simulink model "BiT_Template_pavlo"  (R2025b)
settings: Solver=ode3  StartTime=0.0  StopTime=30  FixedStep=0.005  RelTol=1e-3
StopFcn:
  | user_confirmed = true;
  | disp('Gestoppt?!')
  | 
  | % stop(t);
  | % delete(t);
  | 
  | %% Switch to Config Mode
  | %Tc3_AI.sysManager.ActivateConfiguration();
  | %
  | % Tc3_AI.SwitchToConfig('local')
  | %
  | % %save Solution
  | % Tc3_AI.SaveSolution();
  | %
  | % %% Close Aktive VS Instance
  | % Tc3_AI.closeVsInstance();
libraries: slpidlib x1
settings Model: Creator=clemensm  LastModifiedBy=Felix
settings OptimizationCC: LocalBlockOutputs=off
settings RTWCC: SystemTargetFile=TwinCatGrt.tlc  GenCodeOnly=on  GenerateMakefile=off  TemplateMakefile=tcgrt_msbuild.tmf  TargetLang=C++  Description=TwinCAT GRT Target
settings STFCustomTargetCC: SystemTargetFile=TwinCatGrt.tlc  TargetLangStandard=C++11 (ISO)  CombineOutputUpdateFcns=on  CodeInterfacePackaging=Reusable function  CPPClassGenCompliant=on  GRTInterface=off  GenerateAllocFcn=on  TcCom_DWorkReadOnly=on  TcProject_StaticStlStringCapacity=Auto  TcPlcFb_MonitorExecutionTime=off  TcCom_ContStateCreateSymbols=on  TcProject_IgnorePseudoArrayDimensions=off  TcProject_IncrementVersion=Revision  TcProject_DeployRestart=off  TcProject_UseCodeInfoExporter=on  TcProject_CLanguageStandard=Default  TcCom_VariableSymbolMapping=Identical  TcProject_DrvFileVersion=$<VersionFromFile>  TcProject_ProjectDir=C:\TwinCAT\3.1\CustomConfig\Modules\Ctrl_only  TcProject_DrvProductVersion=$<DrvFileVersion>  TcPlcFb_OemLicenses=$<Project:OemLicenses>  TcCom_OutputCreateSymbols=on  TcCom_TcComWrapperFbProperties=off  TcProject_UseStaticStlString=off  TcProject_PublishTcOSARMv7M=off  TcCom_OnlineChangeRestoreDataAreas=off  TcCom_AllowDataAreaForSharedData=off  TcProject_LibCatPath=$<Project:Dir>\$<Project:Name>.libcat.xml  TcCom_OemLicenses=$<Project:OemLicenses>  TcProject_UseIntrinsics=on  TcCom_ExtendSignalResolution=on  TcCom_ExtModeRtAllowForParameterChange=on  TcProject_UseCodeDescriptor=on  TcProject_SignWithTwinCatCertificate=inherit default  TcProject_GeneratePlcLibrary=off  TcProject_PublishTcOSARMv7A=off  TcProject_PreferIntOverLong=off  TcPlcFb_ExtModeRtAllowExecutionCommands=off  TcProject_Generate=on  TcProject_GenerateStructDutsWithDefaultValues=Auto  TcCom_ExecutionInfoParam=on  TcCom_TcComWrapperFb=off  TcCom_Generate=on  TcProject_PublishParallel=on  TcCom_OutputDataAccess=Output Source DataArea  TcProject_CppLanguageStandard=Default  TcCom_ParametersCreateSymbols=on  TcProject_PublishTcRTx86=on  TcCom_ExecuteModelCode=on  TcPlcFb_UpdateExceptionHandling=CallerExceptions  TcProject_PublishTcRTx64=on  TcCom_OriginalIoBlockNames=off  TcProject_SignTwinCatCertName=MCI_2024_OEM.tccert  TcCom_InputReadOnly=off  TcCom_GroupDisplayName=$<GroupName>  TcProject_PlcVarPrefixes=PVOID=p | BOOL=b | BOOL32=b | DATE=d | TIME_OF_DATE=td | TIME=t | LTIME=t | GUID=n  TcCom_GlobalParamDefaultSharing=Define  TcCom_MonitorExecutionTime=off  TcProject_VersionSrc=$<LatestTMFile>  TcCom_ExecutionSequence=UpdateBeforeOutputMapping  TcCom_InputCreateSymbols=on  TcProject_DataExchangeModulesVersion=$<ModuleGenerator:DataExchange:Version>  TcCom_BlockDiagramVariableAccess=AssignToParent  TcCom_GroupIcon=$<TE140x:Icon>  TcCom_ParametersDataAccess=Internal DataArea  TcProject_LibraryCategories=$<VendorName>  TcProject_CreateUniqueEnumItemNames=off  TcProject_PreferToolArchitectureX64=on  TcProject_PublishPlatformtoolset=Auto  TcCom_InputInitValues=off  TcProject_Description=TwinCAT executable file, generated by TwinCAT $<ModuleGenerator:ProductId>  TcCom_InitExceptionHandling=CallerExceptions  TcCom_DWorkCreateSymbols=on  TcCom_DWorkDataAccess=Internal DataArea  TcProject_GenerateVsSolution=No  TcCom_StepSizeAdaptation=RequireMatchingTaskCycleTime  TcProject_InstallPlcLibrary=off  TcProject_BuildSystem=Auto  TcProject_EnableNewPlatforms=off  TcCom_ExtModeRtWaitForStart=off  TcCom_OutputReadOnly=on  TcCom_ModuleCaller=CyclicTask  TcProject_VendorName=TE140x Module Vendor  TcCom_ModuleIcon=$<TE140x:Icon>  TcCom_BlockIoReadOnly=on  TcProject_UseDescriptorCodeType=on  TcPlcFb_Generate=off  TcCom_ContStateDataAccess=Internal DataArea  TcPlcFb_ExtModeRtAllowForParameterChange=off  TcCom_BlockDiagramExport=on  TcPlcFb_ExtModeRtWaitForStart=off  TcCom_ContStateReadOnly=on  TcProject_Verbosity=Normal  TcProject_UseDataExchangeModules=off  TcProject_PublishTcOSARMv8A=off  TcProject_ClassFactoryName=$<Project:Name>  TcCom_ExecutionInfoOutput=off  TcCom_AccessLockState=Auto  TcCom_InputDataAccess=Input Destination DataArea  TcCom_UpdateExceptionHandling=CallerExceptions  TcCom_TcComWrapperFbPropertyMonitoring=NoMonitoring  TcProject_PublishTcUMx86=off  TcProject_LowestCompatibleTcBuild=$<TwinCAT:Version:BUILD>  TcProject_Versioning=Versioned  TcCom_BlockIoCreateSymbols=on  TcProject_ForceRebuildForPublish=off  TcProject_PublishConfiguration=Release  TcProject_UseTmxExtension=Auto  TcCom_Legacy_ModuleBuildInfoParam=on  TcProject_CreateScopedEnums=Auto  TcProject_VendorIcon=$<TE140x:Icon>  TcCom_ParametersInitValues=on  TcCom_DataStoreDataAccess=None  TcCom_BlockIoDataAccess=Internal DataArea  TcProject_BuildWithWdk=inherit default  TcPlcFb_InitExceptionHandling=CallerExceptions  TcCom_MaxInternalDataAreaParts=5U  TcCom_BlockDiagramDebugInfoExport=on  TcCom_VariableSymbolMappingCustom=$<ModelName>_U=Input|$<ModelName>_Y=Output|$<ModelName>_P=ModelParameters|$<ModelName>_B=BlockIO|$<ModelName>_DW=DWork|$<ModelName>_X=ContStates  TcProject_Copyright=Copyright $<VendorName> $<LocalDateTime:%Y>  TcProject_ProductName=$<ModuleGenerator:ProductId> $<ModuleGenerator:Version:MAJOR.MINOR>  TcCom_ParametersReadOnly=off  TcProject_UseNativeBlockDiagramExport=off  TcProject_Publish=on  TcProject_MaxVisibleArrayElements=200U  TcProject_TmxInstall=on  TcCom_ResolveMaskedSubsystems=on  TcCom_StrictAccessLock=on  TcCom_DataStoreReadOnly=off  TcProject_PublishTcOSx64=off  TcCom_ExtModeRtAllowExecutionCommands=on  TcCom_DataStoreCreateSymbols=on  TcCom_CallerVerification=Default  TcCom_GroupName=TE140x|Simulink Modules  TcProject_PublishTcUMx64=off  TcProject_CoderCppNamespace=coder  TcCom_OnlineChange=off
settings GRTTargetCC: ExtMode=on  ExtModeMexFile=TcExtModeClient  MultiInstanceErrorCode=None  TargetLangStandard=C++11 (ISO)  ParMdlRefBuildCompliant=off  CompOptLevelCompliant=off  MatFileLogging=off  CodeInterfacePackaging=Reusable function  GenerateAllocFcn=on  UseToolchainInfoCompliant=off

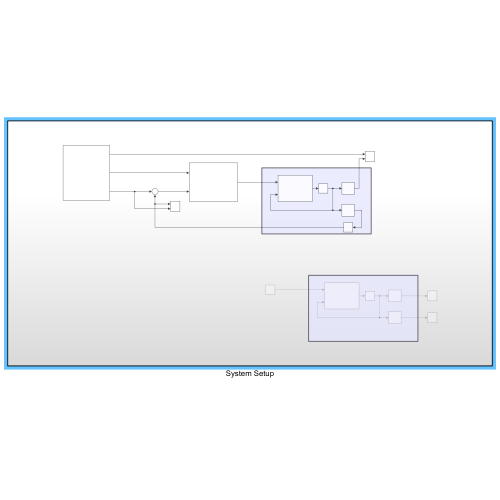
[thumbnail: Simulink's stored preview of the top-level diagram]
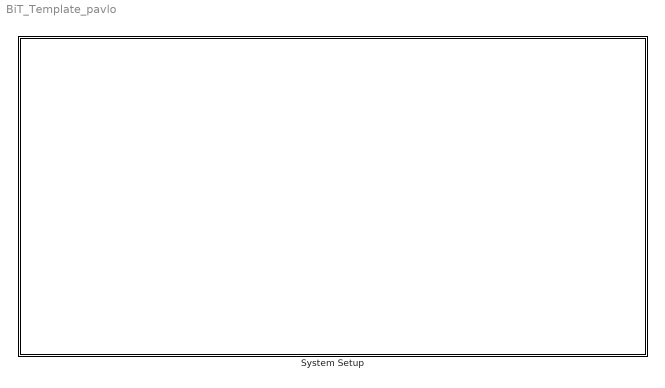
== system BiT_Template_pavlo ==
  System Setup : Subsystem

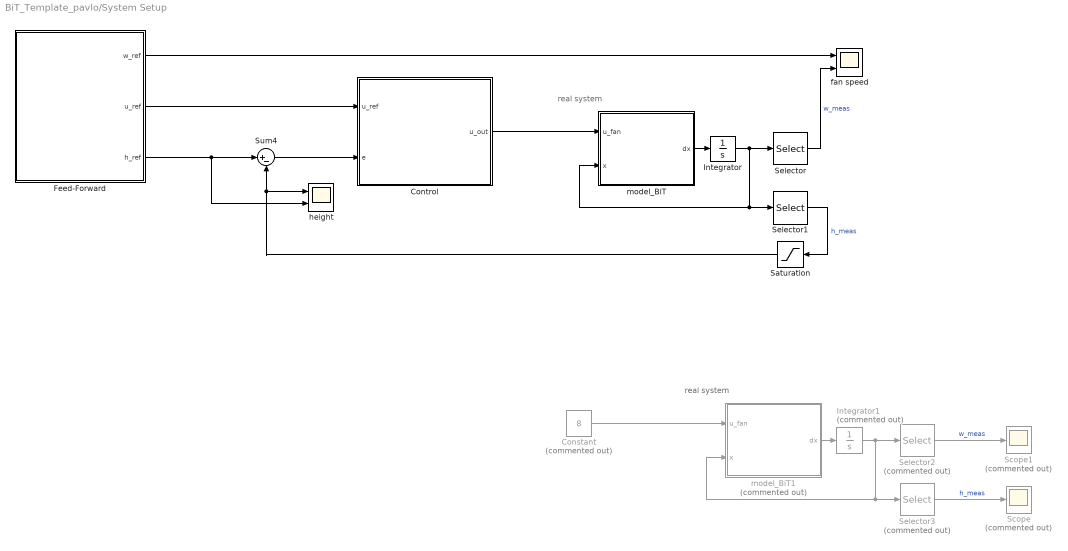
== system BiT_Template_pavlo/System Setup ==
  note: real system
  note: real system
  Constant : Constant  Commented=on  Value=8
  Control : Subsystem
  Feed-Forward : Subsystem
  Integrator : Integrator  InitialCondition=[0.1; 0; 4449]
  Integrator1 : Integrator  Commented=on
  Saturation : Saturate  LowerLimit=0
  Scope : Scope  Commented=on
      settings: ActiveDisplayYMinimum=-4.2397923643804907  ActiveDisplayYMaximum=0.47108804048672109
  Scope1 : Scope  Commented=on
      settings: ActiveDisplayYMinimum=-533.71949992928637  ActiveDisplayYMaximum=4803.4754993635779  DataLoggingVariableName=ScopeData3
  Selector : Selector  InputPortWidth=3  IndexOptions=Index vector (dialog)  Indices=3  OutputSizes=1
  Selector1 : Selector  InputPortWidth=3  IndexOptions=Index vector (dialog)  Indices=1  OutputSizes=1
  Selector2 : Selector  Commented=on  InputPortWidth=3  IndexOptions=Index vector (dialog)  Indices=3  OutputSizes=1
  Selector3 : Selector  Commented=on  InputPortWidth=3  IndexOptions=Index vector (dialog)  Indices=1  OutputSizes=1
  Sum4 : Sum  Inputs=|+-
  fan speed : Scope  NumInputPorts=2
      settings: TimeSpan=60  ActiveDisplayYMinimum=4448.9928221805176  ActiveDisplayYMaximum=4448.9995246053841
  height : Scope  NumInputPorts=2
      settings: TimeSpan=60  ActiveDisplayYMinimum=0.057645230558343891  ActiveDisplayYMaximum=0.32692830771573955  DataLoggingVariableName=ScopeData2
  model_BiT : MATLAB Function  TreatAsAtomicUnit=on
  model_BiT1 : MATLAB Function  Commented=on  TreatAsAtomicUnit=on
  wires:
  Selector1/1 -> Saturation/1  "h_meas"
  Selector/1 -> fan speed/2  "w_meas"
  model_BiT/1(dx) -> Integrator/1
  Integrator/1 -> Selector/1, Selector1/1, model_BiT/2(x)
  Feed-Forward/3(h_ref) -> height/2, Sum4/1
  Feed-Forward/1(w_ref) -> fan speed/1
  Feed-Forward/2(u_ref) -> Control/1(u_ref)
  Sum4/1 -> Control/2(e)
  Control/1(u_out) -> model_BiT/1(u_fan)
  model_BiT1/1(dx) -> Integrator1/1
  Integrator1/1 -> Selector2/1, Selector3/1, model_BiT1/2(x)
  Selector3/1 -> Scope/1  "h_meas"
  Selector2/1 -> Scope1/1  "w_meas"
  Constant/1 -> model_BiT1/1(u_fan)
  Saturation/1 -> height/1, Sum4/2

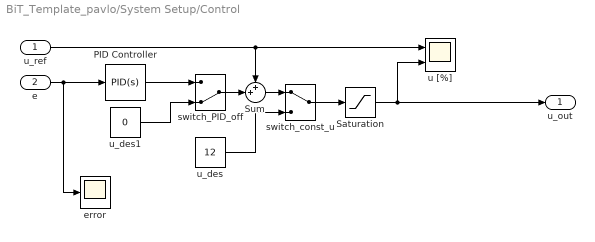
== system BiT_Template_pavlo/System Setup/Control ==
  u_ref : Inport
  e : Inport  Port=2
  PID Controller : slpidlib/PID Controller  Controller=PID  Form=Parallel  TimeDomain=Continuous-time  UseExternalTs=off  SampleTime=-1  IntegratorMethod=Forward Euler  FilterMethod=Forward Euler  ControllerParametersSource=internal  P=58  I=8  UseKiTs=off  D=40  UseExternalDerivativeSource=off  N=123.082708596728  UseFilter=on  TunerSelectOption=Transfer Function Based (PID Tuner App)  InitialConditionSource=internal  InitialConditionForIntegrator=0  InitialConditionForFilter=0  DifferentiatorICPrevScaledInput=0  ExternalReset=none  TrackingMode=off  Kt=1  LimitOutput=off  SatLimitsSource=internal  UpperSaturationLimit=inf  LowerSaturationLimit=-inf  LinearizeAsGain=on  AntiWindupMode=none  Kb=1  LimitIntegrator=off  UpperIntegratorSaturationLimit=inf  LowerIntegratorSaturationLimit=-inf  POutMin=[]  POutMax=[]  IOutMin=[]  IOutMax=[]  DOutMin=[]  DOutMax=[]  NOutMin=[]  NOutMax=[]  SumOutMin=[]  SumOutMax=[]  SaturationOutMin=[]  SaturationOutMax=[]  PParamMin=[]  PParamMax=[]  IParamMin=[]  IParamMax=[]  DParamMin=[]  DParamMax=[]  NParamMin=[]  NParamMax=[]  KbParamMin=[]  KbParamMax=[]  KtParamMin=[]  KtParamMax=[]  KbOutMin=[]  KbOutMax=[]  KtOutMin=[]  KtOutMax=[]  IntegratorOutMin=[]  IntegratorOutMax=[]  FilterOutMin=[]  FilterOutMax=[]  SumI1OutMin=[]  SumI1OutMax=[]  SumI2OutMin=[]  SumI2OutMax=[]  SumI3OutMin=[]  SumI3OutMax=[]  SumI4OutMin=[]  SumI4OutMax=[]  SumDOutMin=[]  SumDOutMax=[]  DifferentiatorOutMin=[]  DifferentiatorOutMax=[]  FilterDiffOutCoefMin=[]  FilterDiffOutCoefMax=[]  ReciprocalOutMin=[]  ReciprocalOutMax=[]  SumDenOutMin=[]  SumDenOutMax=[]  SumNumOutMin=[]  SumNumOutMax=[]  DivideOutMin=[]  DivideOutMax=[]  UdiffTsProdOutMin=[]  UdiffTsProdOutMax=[]  NTsProdOutMin=[]  NTsProdOutMax=[]  UintegralTsProdOutMin=[]  UintegralTsProdOutMax=[]  UngainTsProdOutMin=[]  UngainTsProdOutMax=[]  ClampingZeroOutDataTypeStr=Inherit: Inherit via back propagation  ClampingZeroOutMin=[]  ClampingZeroOutMax=[]  FilterDenConstantOutDataTypeStr=Inherit: Inherit via back propagation  FilterDenConstantOutMin=[]  FilterDenConstantOutMax=[]  PCopyOutDataTypeStr=Inherit: Inherit via back propagation  PCopyOutMin=[]  PCopyOutMax=[]  NCopyOutDataTypeStr=Inherit: Inherit via back propagation  NCopyOutMin=[]  NCopyOutMax=[]  IntegratorContinuousStateAttributes=''  IntegratorStateMustResolveToSignalObject=off  IntegratorRTWStateStorageClass=Auto  FilterContinuousStateAttributes=''  FilterStateMustResolveToSignalObject=off  FilterRTWStateStorageClass=Auto  ParallelPVariant=InternalParameters  IdealPVariant=Disabled  IVariant=InternalParameters  DVariant=InternalParameters  IntegratorVariant=Continuous  SatVariant=Disabled  AWVariant=Passthrough  PCopyVariant=Disabled  TRVariant=Disabled  FdbkBlocksVariant=Forward  IdealPFdbkVariant=Disabled  SatFdbkVariant=Disabled  DerivativeFilterVariant=ContFilter  NVariant=InternalParameters  NCopyVariant=Disabled  FilterICVariant=InternalICsFilter  IntegratorICVariant=InternalICs  ExternalResetVariant=Disabled  TRSumVariant=Passthrough  SumFdbkVariant=Disabled  SumVariant=Sum_PID  TsampFilterVariant=InternalTs  TsampNgainVariant=Passthrough  TsampIntegralVariant=Disabled_SignalSpec  ExternalSaturationOutDataTypeStr=Inherit: Same as second input  DerivativeSourceVariant=ErrorSignal  PreIntVariant=InternalPreInt
  Saturation : Saturate  UpperLimit=100  LowerLimit=0
  Sum : Sum  Inputs=++|
  error : Scope
      settings: ActiveDisplayYMinimum=-1  ActiveDisplayYMaximum=1  DataLoggingVariableName=ScopeData4
  switch_PID_off : ManualSwitch  CurrentSetting=0
  switch_const_u : ManualSwitch
  u [%] : Scope  NumInputPorts=2
      settings: TimeSpan=60  ActiveDisplayYMinimum=2.2902737072273522  ActiveDisplayYMaximum=10.951910082492102
  u_des : Constant  Value=12
  u_des1 : Constant  Value=0
  u_out : Outport
  wires:
  u_des/1 -> switch_const_u/2
  Saturation/1 -> u_out/1, u [%]/2
  e/1 -> error/1, PID Controller/1
  switch_const_u/1 -> Saturation/1
  u_ref/1 -> u [%]/1, Sum/1
  Sum/1 -> switch_const_u/1
  PID Controller/1 -> switch_PID_off/1
  switch_PID_off/1 -> Sum/2
  u_des1/1 -> switch_PID_off/2

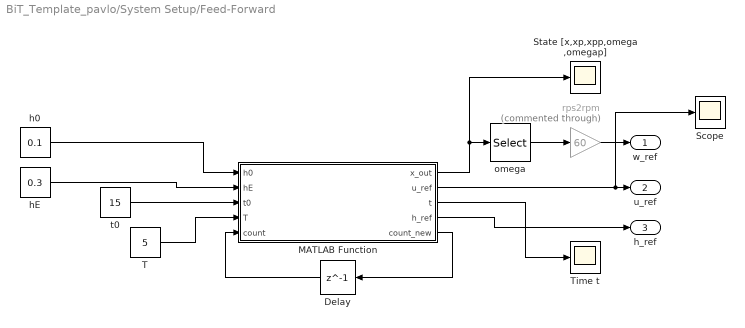
== system BiT_Template_pavlo/System Setup/Feed-Forward ==
  Delay : Delay  DelayLength=1
  MATLAB Function : MATLAB Function  TreatAsAtomicUnit=on
  Scope : Scope
      settings: ActiveDisplayYMinimum=5.5436516329969319  ActiveDisplayYMaximum=10.495149818555896  DataLoggingVariableName=ScopeData5
  State [x,xp,xpp,omega,omegap] : Scope
      settings: TimeSpan=60  ActiveDisplayYMinimum=0.075000000000000011  ActiveDisplayYMaximum=0.32499999999999996
  T : Constant  Value=5
  Time t : Scope
      settings: ActiveDisplayYMinimum=-1  ActiveDisplayYMaximum=1
  h0 : Constant  Value=0.1
  hE : Constant  Value=0.3
  omega : Selector  InputPortWidth=5  IndexOptions=Index vector (dialog)  Indices=4  OutputSizes=1
  rps2rpm : Gain  Commented=through  Gain=60
  t0 : Constant  Value=15
  w_ref : Outport
  u_ref : Outport  Port=2
  h_ref : Outport  Port=3
  wires:
  h0/1 -> MATLAB Function/1(h0)
  omega/1 -> rps2rpm/1
  MATLAB Function/3(t) -> Time t/1
  T/1 -> MATLAB Function/4(T)
  t0/1 -> MATLAB Function/3(t0)
  Delay/1 -> MATLAB Function/5(count)
  MATLAB Function/5(count_new) -> Delay/1
  hE/1 -> MATLAB Function/2(hE)
  MATLAB Function/1(x_out) -> State [x,xp,xpp,omega,omegap]/1, omega/1
  MATLAB Function/2(u_ref) -> Scope/1, u_ref/1
  rps2rpm/1 -> w_ref/1
  MATLAB Function/4(h_ref) -> h_ref/1

== matlab function BiT_Template_pavlo/System Setup/model_BiT ==
  data: u_fan input; dx output; x input
function dx  = model_BiT(u_fan,x)
% model_BiT represents the differential equations of the ball in tube test
% rig

% u_fan ... duty cycle in [%]
% x[3] ... state that includes
%       x1 = h ... height of the ball in [m]
%       x2 = dh ... change of heihgt of the ball in [m/s]
%       x3 = w ... fan speed in [rpm]

u0 = -33;
alpha1 = 0.000745736;
alpha2 = 0.148139;
alpha3 = 9.81;
tau_omega = 1.965; 
k_omega = 97.8373;

dx1 = x(2);
dx2 = (alpha1*x(3) - alpha2*x(2))^2 - alpha3;
dx3 = (k_omega * (u_fan - u0) - x(3)) / tau_omega;

dx = [dx1; dx2; dx3];

== matlab function BiT_Template_pavlo/System Setup/Feed-Forward/MATLAB Function ==
  data: x_out output; u_ref output; h0 input; hE input; t0 input; T input; t output; h_ref output; count input; count_new output
function [x_out,u_ref,t,h_ref,count_new] = feed_forward(h0,hE,t0,T,count)

count_new = count+1;
dT = 0.005;
t_total = count_new*dT;

n = floor(t_total/(t0 + T));
t = rem(t_total, (t0+T));


u0 = -33;
alpha1 = 0.000745736;
alpha2 = 0.148139;
alpha3 = 9.81;
tau_omega = 1.965; 
k_omega = 97.8373;

xp_ref = 0;
xpp_ref = 0;
xppp_ref = 0;

if t<t0
    if rem(n, 2) == 0
        x_ref = h0;
    else
        x_ref = hE;
    end
elseif t>t0+T
    if rem(n, 2) == 0
        x_ref = hE;
    else
        x_ref = h0;
    end
else
    s = (t - t0)/T;
    x_ref = h0 - (h0 - hE) * (35*s.^4-84*s.^5 +70*s.^6 - 20*s.^7);
    xp_ref = -(h0 - hE) * (140*s.^3 - 420*s.^4 + 420*s.^5 - 140*s.^6) / T;
    xpp_ref = -(h0 - hE) * (420*s.^2 - 1680*s.^3 + 2100*s.^4 - 840*s.^5) / T^2;
    xppp_ref = -(h0 - hE) * (840*s - 5040*s.^2 + 8400*s.^3 - 4200*s.^4)/T^3;
end

acc = xpp_ref + alpha3;

omega = (sqrt(acc) + alpha2 * xp_ref) / alpha1;
omega_p = (xppp_ref/(2*sqrt(acc)) + alpha2*xpp_ref)/alpha1;

u = (tau_omega*omega_p + omega)/k_omega + u0;

h_ref = x_ref;

u_min = 0;
u_max = 100;
u = max(min(u, u_max), u_min);

u_ref = u; 
x_out = [x_ref,xp_ref,xpp_ref,omega,omega_p]';
end

== matlab function BiT_Template_pavlo/System Setup/model_BiT1 ==
  data: u_fan input; dx output; x input
function dx  = model_BiT(u_fan,x)
% model_BiT represents the differential equations of the ball in tube test
% rig

% u_fan ... duty cycle in [%]
% x[3] ... state that includes
%       x1 = h ... height of the ball in [m]
%       x2 = dh ... change of heihgt of the ball in [m/s]
%       x3 = w ... fan speed in [rpm]
alpha_1 = 7.04 * 10^-4;
alpha_2 = 0.92;
alpha_3 = 9.81;
K_t = 112.362;
u0 = -33;
tau = 1.319;


dx1 = x(2);
dx2 = (alpha_1*x(3) - alpha_2*x(2))^2 - alpha_3;
dx3 = (K_t * (u_fan - u0) - x(3)) / tau;

dx = [dx1; dx2; dx3];
